simulink model "CruiseControl_r2014a"  (R2018a)
settings: Solver=ode45  StartTime=0.0  StopTime=40.0  MaxStep=1e-2  RelTol=1e-3
values from neighbouring files (symbols this model uses):
  a = sortsolution(11,2)    [example_8_2.m]
  m = max(y)    [example_8_2.m]
undefined symbols (not defined in the file or in its folder): b, g
settings Model: Creator=jofr  LastModifiedBy=rodralez
settings DataIOCC: LimitDataPoints=on  SaveFormat=Array  SignalLoggingSaveFormat=ModelDataLogs
settings OptimizationCC: BlockReduction=off  BooleanDataType=off  LifeSpan=inf
settings DebuggingCC: SaveWithParameterizedLinksMsg=none  UnderspecifiedInitializationDetection=Classic  MergeDetectMultiDrivingBlocksExec=none  SignalResolutionControl=TryResolveAllWithWarning  MultiTaskDSMMsg=warning  MultiTaskCondExecSysMsg=none  SFUnexpectedBacktrackingDiag=warning  SFNoUnconditionalDefaultTransitionDiag=warning  SFExecutionAtInitializationDiag=none
settings HardwareCC: ProdBitPerPointer=32  ProdBitPerSizeT=32  ProdBitPerPtrDiffT=32  ProdLargestAtomicFloat=None  ProdIntDivRoundTo=Undefined  ProdEndianess=Unspecified  ProdWordSize=32  ProdHWDeviceType=32-bit Generic  TargetUnknown=on
settings ModelReferenceCC: PropagateSignalLabelsOutOfModel=off
settings CodeAppCC: StateflowObjectComments=on
settings GRTTargetCC: TargetLangStandard=C89/C90 (ANSI)  GeneratePreprocessorConditionals=Disable all
settings ConfigComp: CovMetricSettings=dw  CovHtmlReporting=on  CovSaveCumulativeToWorkspaceVar=on  CovSaveSingleToWorkspaceVar=on  CovExternalEMLEnable=off

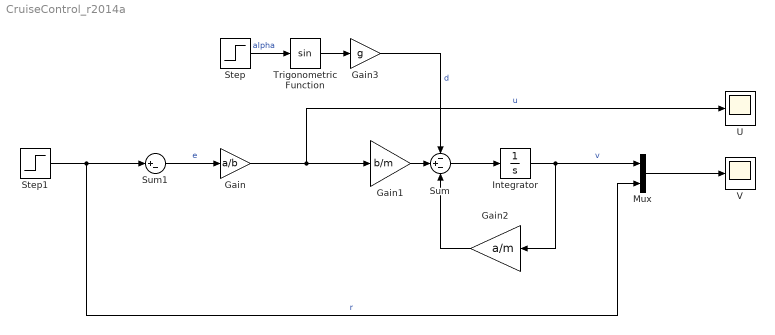
== system CruiseControl_r2014a ==
  Gain : Gain  Gain=a/b
  Gain1 : Gain  Gain=b/m
  Gain2 : Gain  Gain=a/m
  Gain3 : Gain  Gain=g
  Integrator : Integrator  InitialCondition=25
  Mux : Mux  Inputs=2
  Step : Step  Time=20  After=2*pi/180  SampleTime=0
  Step1 : Step  Time=10  Before=25  After=30  SampleTime=0
  Sum : Sum  Inputs=-+-
  Sum1 : Sum  Inputs=|+-
  Trigonometric Function : Trigonometry
  U : Scope
  V : Scope
  wires:
  Gain2/1 -> Sum/3
  Gain1/1 -> Sum/2
  Trigonometric Function/1 -> Gain3/1
  Sum/1 -> Integrator/1
  Step/1 -> Trigonometric Function/1  "alpha"
  Integrator/1 -> Mux/1, Gain2/1  "v"
  Sum1/1 -> Gain/1  "e"
  Step1/1 -> Mux/2, Sum1/1  "r"
  Gain/1 -> Gain1/1, U/1  "u"
  Mux/1 -> V/1
  Gain3/1 -> Sum/1  "d"
